simulink model "week3_inclass_ACC_v_1_1"  (R2020b)
settings: Solver=FixedStepAuto  StartTime=0.0  StopTime=500  RelTol=1e-3
undefined symbols (not defined in the file or in its folder): sigbuilder_block
libraries: simulink x3, pid_lib x2
settings Model: Creator=anime  LastModifiedBy=anime

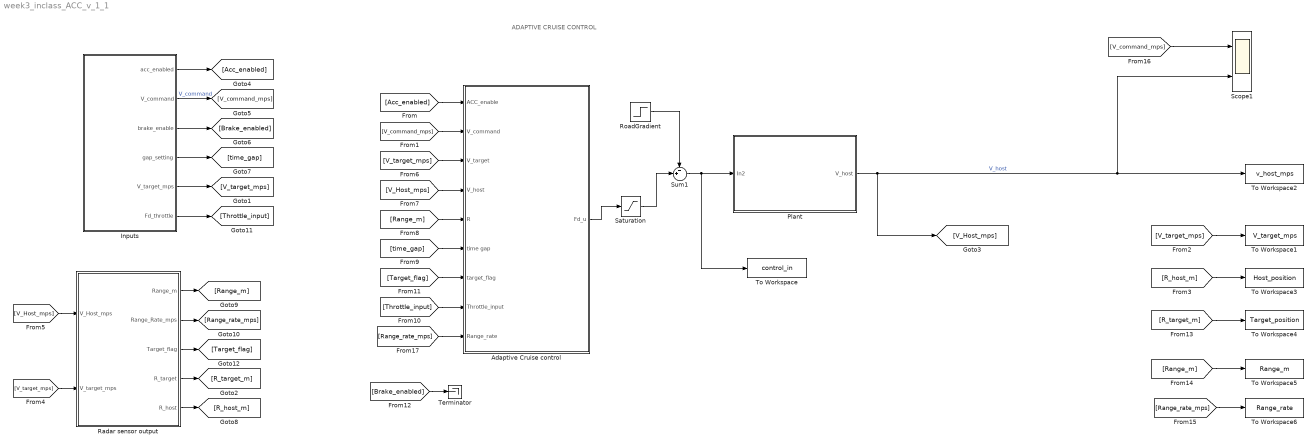
== system week3_inclass_ACC_v_1_1 ==
  note: ADAPTIVE CRUISE CONTROL
  Adaptive Cruise control : Subsystem
  Inputs : Subsystem
  Plant : Subsystem
  Radar sensor output : Subsystem
  RoadGradient : Step  Time=500  After=200  SampleTime=0
  Saturation : Saturate  UpperLimit=1000  LowerLimit=-1000
  Scope1 : Scope  NumInputPorts=2
  Sum1 : Sum  Inputs=-+|
  Terminator : Terminator
  To Workspace : ToWorkspace  VariableName=control_in  SampleTime=-1
  To Workspace1 : ToWorkspace  VariableName=V_target_mps  SampleTime=-1
  To Workspace2 : ToWorkspace  VariableName=v_host_mps  SampleTime=-1
  To Workspace3 : ToWorkspace  VariableName=Host_position  SampleTime=-1
  To Workspace4 : ToWorkspace  VariableName=Target_position  SampleTime=-1
  To Workspace5 : ToWorkspace  VariableName=Range_m  SampleTime=-1
  To Workspace6 : ToWorkspace  VariableName=Range_rate  SampleTime=-1
  wires:
  Adaptive Cruise control/1(Fd_u) -> Saturation/1
  Saturation/1 -> Sum1/2
  RoadGradient/1 -> Sum1/1
  Sum1/1 -> Plant/1(In2), To Workspace/1
  Plant/1(V_host) -> [V_Host_mps], Scope1/2, To Workspace2/1  "V_host"
  Inputs/1(acc_enabled) -> [Acc_enabled]
  Inputs/2(V_command) -> [V_command_mps]  "V_command"
  Inputs/6(Fd_throttle) -> [Throttle_input]
  Inputs/5(V_target_mps) -> [V_target_mps]
  Inputs/4(gap_setting) -> [time_gap]
  Inputs/3(brake_enable) -> [Brake_enabled]
  [V_command_mps] -> Adaptive Cruise control/2(V_command)
  [V_target_mps] -> Adaptive Cruise control/3(V_target)
  [V_Host_mps] -> Adaptive Cruise control/4(V_host)
  [time_gap] -> Adaptive Cruise control/6(time gap)
  [V_Host_mps] -> Radar sensor output/1(V_Host_mps)
  [V_target_mps] -> Radar sensor output/2(V_target_mps)
  Radar sensor output/1(Range_m) -> [Range_m]
  Radar sensor output/2(Range_Rate_mps) -> [Range_rate_mps]
  Radar sensor output/3(Target_flag) -> [Target_flag]
  [Range_m] -> Adaptive Cruise control/5(R)
  [Acc_enabled] -> Adaptive Cruise control/1(ACC_enable)
  [Target_flag] -> Adaptive Cruise control/7(target_flag)
  [Throttle_input] -> Adaptive Cruise control/8(Throttle_input)
  [Brake_enabled] -> Terminator/1
  Radar sensor output/4(R_target) -> [R_target_m]
  Radar sensor output/5(R_host) -> [R_host_m]
  [V_target_mps] -> To Workspace1/1
  [R_host_m] -> To Workspace3/1
  [R_target_m] -> To Workspace4/1
  [Range_m] -> To Workspace5/1
  [Range_rate_mps] -> To Workspace6/1
  [V_command_mps] -> Scope1/1
  [Range_rate_mps] -> Adaptive Cruise control/9(Range_rate)

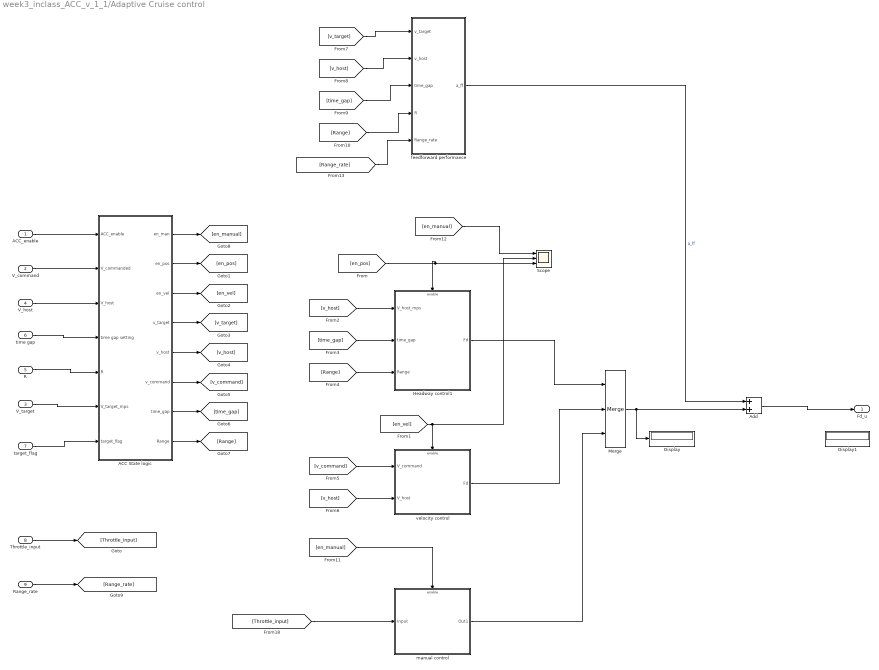
== system week3_inclass_ACC_v_1_1/Adaptive Cruise control ==
  ACC_enable : Inport
  V_command : Inport  Port=2
  V_target : Inport  Port=3
  V_host : Inport  Port=4
  R : Inport  Port=5
  time gap : Inport  Port=6
  target_flag : Inport  Port=7
  Throttle_input : Inport  Port=8
  Range_rate : Inport  Port=9
  ACC State logic : Subsystem
  Add : Sum
  Display : Display
  Display1 : Display
  Headway control1 : Subsystem
  Merge : Merge  Inputs=3
  Scope : Scope  NumInputPorts=3
  feedforward performance : Subsystem
  manual control : Subsystem
  velocity control : Subsystem
  Fd_u : Outport
  wires:
  [en_pos] -> Headway control1/Enable, Scope/3
  [en_vel] -> velocity control/Enable, Scope/2
  [time_gap] -> Headway control1/2(time_gap)
  [Range] -> Headway control1/3(Range)
  [v_command] -> velocity control/1(V_command)
  [v_host] -> velocity control/2(V_host)
  Headway control1/1(Fd) -> Merge/1
  velocity control/1(Fd) -> Merge/2
  [en_manual] -> manual control/Enable
  manual control/1(Out1) -> Merge/3
  [en_manual] -> Scope/1
  [Throttle_input] -> manual control/1(Input)
  ACC State logic/5(v_host) -> [v_host]
  ACC State logic/6(v_command) -> [v_command]
  ACC State logic/4(v_target) -> [v_target]
  ACC State logic/8(Range) -> [Range]
  V_host/1 -> ACC State logic/3(V_host)
  ACC State logic/7(time_gap) -> [time_gap]
  V_command/1 -> ACC State logic/2(V_commanded)
  R/1 -> ACC State logic/5(R)
  ACC_enable/1 -> ACC State logic/1(ACC_enable)
  ACC State logic/1(en_man) -> [en_manual]
  ACC State logic/2(en_pos) -> [en_pos]
  V_target/1 -> ACC State logic/6(V_target_mps)
  ACC State logic/3(en_vel) -> [en_vel]
  time gap/1 -> ACC State logic/4(time gap setting)
  target_flag/1 -> ACC State logic/7(target_flag)
  Throttle_input/1 -> [Throttle_input]
  [v_host] -> Headway control1/1(V_host_mps)
  Merge/1 -> Add/2, Display/1
  Range_rate/1 -> [Range_rate]
  Add/1 -> Fd_u/1
  [v_target] -> feedforward performance/1(v_target)
  [Range_rate] -> feedforward performance/5(Range_rate)
  [v_host] -> feedforward performance/2(v_host)
  [time_gap] -> feedforward performance/3(time_gap)
  [Range] -> feedforward performance/4(R)
  feedforward performance/1(a_ff) -> Add/1  "a_ff"

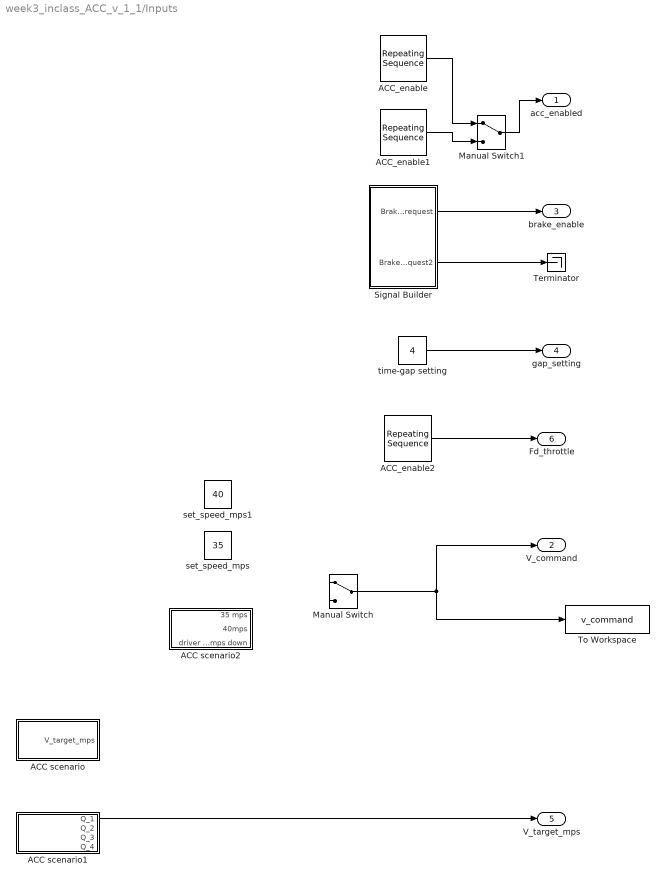
== system week3_inclass_ACC_v_1_1/Inputs ==
  ACC scenario : Subsystem  Tag=STV Subsys  LoadFcn=sigbuilder_block('load');  StartFcn=sigbuilder_block('start');  StopFcn=sigbuilder_block('stop');  ClipboardFcn=sigbuilder_block('clipboard');  mask(Sigbuilder block){tuvar=[0:10]}
      mask help: Simulink:masks:SigbuilderBlock_MD
      mask init:
      | if ~strcmp(get_param(bdroot(gcbh),'SimulationStatus'),'stopped') tuvar = sigbuilder_block('maskInit'); end
      settings: CopyFcn=sigbuilder_block('copy');  DeleteFcn=sigbuilder_block('delete');  ModelCloseFcn=sigbuilder_block('modelClose');  PreSaveFcn=sigbuilder_block('preSave');  PauseFcn=sigbuilder_block('pause');  ContinueFcn=sigbuilder_block('continue');  NameChangeFcn=sigbuilder_block('namechange');  OpenFcn=sigbuilder_block('open',[5.4 44.4 1141.2 541.8 ]);  CloseFcn=sigbuilder_block('close');
      mask Display: plot(0, 0, 100, 100,[2, 2, 32, 32, 2], [68, 8, 8, 68, 68],[32, 2], [38, 38], [32, 19, 2],[53, 60, 44], [32, 17, 17, 2],[16, 16, 31, 31]);txt = getActiveGroup(gcbh);text(2, 100, txt,'verticalAlignment', 'top');
  ACC scenario1 : Subsystem  Tag=STV Subsys  LoadFcn=sigbuilder_block('load');  StartFcn=sigbuilder_block('start');  StopFcn=sigbuilder_block('stop');  ClipboardFcn=sigbuilder_block('clipboard');  mask(Sigbuilder block){tuvar=[0:10]}
      mask help: Simulink:masks:SigbuilderBlock_MD
      mask init:
      | if ~strcmp(get_param(bdroot(gcbh),'SimulationStatus'),'stopped') tuvar = sigbuilder_block('maskInit'); end
      settings: CopyFcn=sigbuilder_block('copy');  DeleteFcn=sigbuilder_block('delete');  ModelCloseFcn=sigbuilder_block('modelClose');  PreSaveFcn=sigbuilder_block('preSave');  PauseFcn=sigbuilder_block('pause');  ContinueFcn=sigbuilder_block('continue');  NameChangeFcn=sigbuilder_block('namechange');  OpenFcn=sigbuilder_block('open',[12.75 109.5 1141.5 542.25 ]);  CloseFcn=sigbuilder_block('close');
      mask Display: plot(0, 0, 100, 100,[2, 2, 32, 32, 2], [68, 8, 8, 68, 68],[32, 2], [38, 38], [32, 19, 2],[53, 60, 44], [32, 17, 17, 2],[16, 16, 31, 31]);txt = getActiveGroup(gcbh);text(2, 100, txt,'verticalAlignment', 'top');
  ACC scenario2 : Subsystem  Tag=STV Subsys  LoadFcn=sigbuilder_block('load',[5.4 44.4 1141.2 541.8 ]);  StartFcn=sigbuilder_block('start');  StopFcn=sigbuilder_block('stop');  ClipboardFcn=sigbuilder_block('clipboard');  mask(Sigbuilder block){tuvar=[0:10]}
      mask help: Simulink:masks:SigbuilderBlock_MD
      mask init:
      | if ~strcmp(get_param(bdroot(gcbh),'SimulationStatus'),'stopped') tuvar = sigbuilder_block('maskInit'); end
      settings: CopyFcn=sigbuilder_block('copy');  DeleteFcn=sigbuilder_block('delete');  ModelCloseFcn=sigbuilder_block('modelClose');  PreSaveFcn=sigbuilder_block('preSave');  PauseFcn=sigbuilder_block('pause');  ContinueFcn=sigbuilder_block('continue');  NameChangeFcn=sigbuilder_block('namechange');  OpenFcn=sigbuilder_block('open',[5.4 44.4 1141.2 541.8 ]);  CloseFcn=sigbuilder_block('close');
      mask Display: plot(0, 0, 100, 100,[2, 2, 32, 32, 2], [68, 8, 8, 68, 68],[32, 2], [38, 38], [32, 19, 2],[53, 60, 44], [32, 17, 17, 2],[16, 16, 31, 31]);txt = getActiveGroup(gcbh);text(2, 100, txt,'verticalAlignment', 'top');
  ACC_enable : simulink/Sources/Repeating Sequence  rep_seq_t=[0 25 50 75 100 125 150 175 200 250 300 350 400 450 500 550 600 650 700]  rep_seq_y=[1 1 1 1 1 1 1 1 1 1 1 1 1 1 1 1 1 1 1]
  ACC_enable1 : simulink/Sources/Repeating Sequence  rep_seq_t=[0 25 50 75 100 125 150 175 200 250 300 350 400 450 500 550 600 650 700]  rep_seq_y=[1 1 1 1 1 1 1 1 1 0 0 0 0 0 0 1 1 1 1]
  ACC_enable2 : simulink/Sources/Repeating Sequence  rep_seq_t=[0 25 50 75 100 125 150 175 200 250 300 350 400 450 500 550 600 650 700]  rep_seq_y=[1 1 1 1 1 1 1 1 1 1 1 1 1 1 1 1 1 1 1]*0
  Manual Switch : ManualSwitch
  Manual Switch1 : ManualSwitch
  Signal Builder : Subsystem  Tag=STV Subsys  LoadFcn=sigbuilder_block('load');  StartFcn=sigbuilder_block('start');  StopFcn=sigbuilder_block('stop');  ClipboardFcn=sigbuilder_block('clipboard');  mask(Sigbuilder block){tuvar=[0:10]}
      mask help: Simulink:masks:SigbuilderBlock_MD
      mask init:
      | if ~strcmp(get_param(bdroot(gcbh),'SimulationStatus'),'stopped') tuvar = sigbuilder_block('maskInit'); end
      settings: CopyFcn=sigbuilder_block('copy');  DeleteFcn=sigbuilder_block('delete');  ModelCloseFcn=sigbuilder_block('modelClose');  PreSaveFcn=sigbuilder_block('preSave');  PauseFcn=sigbuilder_block('pause');  ContinueFcn=sigbuilder_block('continue');  NameChangeFcn=sigbuilder_block('namechange');  OpenFcn=sigbuilder_block('open',[305.4 42.6 814.8 400.2 ]);  CloseFcn=sigbuilder_block('close');
      mask Display: plot(0, 0, 100, 100,[2, 2, 32, 32, 2], [68, 8, 8, 68, 68],[32, 2], [38, 38], [32, 19, 2],[53, 60, 44], [32, 17, 17, 2],[16, 16, 31, 31]);txt = getActiveGroup(gcbh);text(2, 100, txt,'verticalAlignment', 'top');
  Terminator : Terminator
  To Workspace : ToWorkspace  VariableName=v_command  SampleTime=-1
  set_speed_mps : Constant  Value=35
  set_speed_mps1 : Constant  Value=40
  time-gap setting : Constant  Value=4
  acc_enabled : Outport
  V_command : Outport  Port=2
  brake_enable : Outport  Port=3
  gap_setting : Outport  Port=4
  V_target_mps : Outport  Port=5
  Fd_throttle : Outport  Port=6
  wires:
  Signal Builder/1(Brake_request) -> brake_enable/1
  time-gap setting/1 -> gap_setting/1
  Signal Builder/2(Brake_request2) -> Terminator/1
  ACC_enable2/1 -> Fd_throttle/1
  Manual Switch/1 -> V_command/1, To Workspace/1
  ACC_enable/1 -> Manual Switch1/1
  Manual Switch1/1 -> acc_enabled/1
  ACC_enable1/1 -> Manual Switch1/2
  ACC scenario1/1(Q_1) -> V_target_mps/1

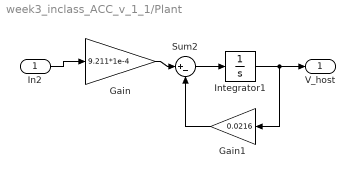
== system week3_inclass_ACC_v_1_1/Plant ==
  In2 : Inport
  Gain : Gain  Gain=9.211*1e-4
  Gain1 : Gain  Gain=0.0216
  Integrator1 : Integrator  InitialCondition=25
  Sum2 : Sum  Inputs=|+-
  V_host : Outport  VectorParamsAs1DForOutWhenUnconnected=off
  wires:
  Gain1/1 -> Sum2/2
  Integrator1/1 -> Gain1/1, V_host/1
  Gain/1 -> Sum2/1
  Sum2/1 -> Integrator1/1
  In2/1 -> Gain/1

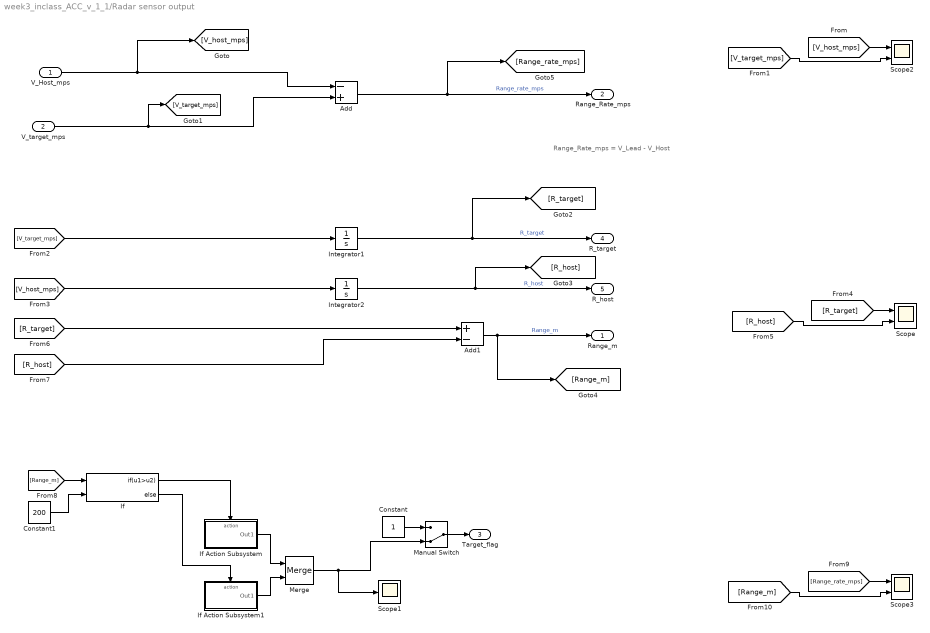
== system week3_inclass_ACC_v_1_1/Radar sensor output ==
  note: Range_Rate_mps = V_Lead - V_Host
  V_Host_mps : Inport
  V_target_mps : Inport  Port=2
  Add : Sum  Inputs=-+
  Add1 : Sum  Inputs=+-
  Constant : Constant
  Constant1 : Constant  Value=200
  If : If  NumInputs=2  IfExpression=u1>u2
  If Action Subsystem : Subsystem  TreatAsAtomicUnit=on
  If Action Subsystem1 : Subsystem  TreatAsAtomicUnit=on
  Integrator1 : Integrator  InitialCondition=500
  Integrator2 : Integrator
  Manual Switch : ManualSwitch  CurrentSetting=0
  Merge : Merge
  Scope : Scope  NumInputPorts=2
  Scope1 : Scope
  Scope2 : Scope  NumInputPorts=2
  Scope3 : Scope  NumInputPorts=2
  Range_m : Outport
  Range_Rate_mps : Outport  Port=2
  Target_flag : Outport  Port=3
  R_target : Outport  Port=4
  R_host : Outport  Port=5
  wires:
  V_target_mps/1 -> Add/2, [V_target_mps]
  V_Host_mps/1 -> Add/1, [V_host_mps]
  Add/1 -> [Range_rate_mps], Range_Rate_mps/1  "Range_rate_mps"
  Integrator1/1 -> [R_target], R_target/1  "R_target"
  Integrator2/1 -> [R_host], R_host/1  "R_host"
  Add1/1 -> [Range_m], Range_m/1  "Range_m"
  Constant/1 -> Manual Switch/1
  Manual Switch/1 -> Target_flag/1
  If/1 -> If Action Subsystem/Action
  If/2 -> If Action Subsystem1/Action
  If Action Subsystem/1(Out1) -> Merge/1
  If Action Subsystem1/1(Out1) -> Merge/2
  Merge/1 -> Scope1/1, Manual Switch/2
  Constant1/1 -> If/2
  [V_host_mps] -> Scope2/1
  [V_target_mps] -> Scope2/2
  [V_target_mps] -> Integrator1/1
  [V_host_mps] -> Integrator2/1
  [R_target] -> Scope/1
  [R_host] -> Scope/2
  [R_target] -> Add1/1
  [R_host] -> Add1/2
  [Range_m] -> If/1
  [Range_rate_mps] -> Scope3/1
  [Range_m] -> Scope3/2

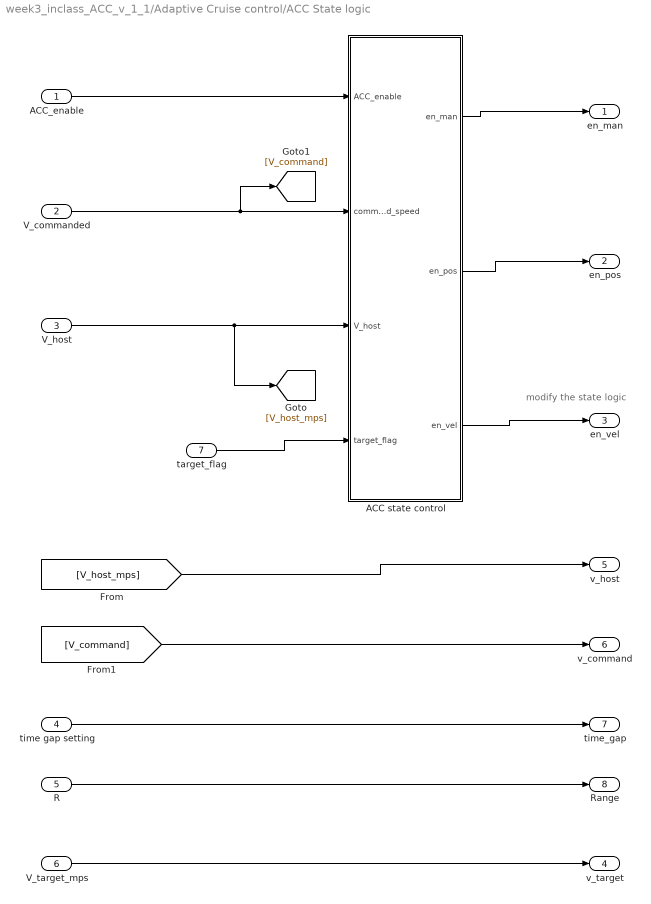
== system week3_inclass_ACC_v_1_1/Adaptive Cruise control/ACC State logic ==
  note: modify the state logic
  ACC_enable : Inport
  V_commanded : Inport  Port=2
  V_host : Inport  Port=3
  time gap setting : Inport  Port=4
  R : Inport  Port=5
  V_target_mps : Inport  Port=6
  target_flag : Inport  Port=7
  ACC state control : Stateflow chart  TreatAsAtomicUnit=on
  en_man : Outport
  en_pos : Outport  Port=2
  en_vel : Outport  Port=3
  v_target : Outport  Port=4
  v_host : Outport  Port=5
  v_command : Outport  Port=6
  time_gap : Outport  Port=7
  Range : Outport  Port=8
  wires:
  ACC state control/1(en_man) -> en_man/1
  ACC state control/2(en_pos) -> en_pos/1
  ACC state control/3(en_vel) -> en_vel/1
  ACC_enable/1 -> ACC state control/1(ACC_enable)
  V_commanded/1 -> [V_command], ACC state control/2(commanded_speed)
  V_target_mps/1 -> v_target/1
  V_host/1 -> [V_host_mps], ACC state control/3(V_host)
  target_flag/1 -> ACC state control/4(target_flag)
  [V_host_mps] -> v_host/1
  [V_command] -> v_command/1
  time gap setting/1 -> time_gap/1
  R/1 -> Range/1

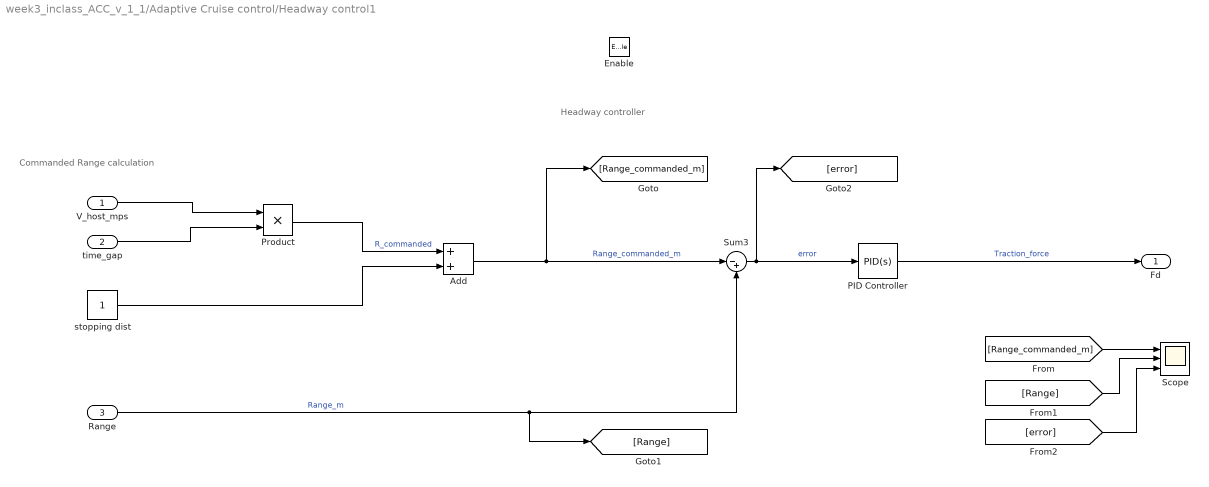
== system week3_inclass_ACC_v_1_1/Adaptive Cruise control/Headway control1 ==
  note: Commanded Range calculation
  note: Headway controller
  V_host_mps : Inport
  time_gap : Inport  Port=2
  Range : Inport  Port=3
  Enable : EnablePort
  Add : Sum
  PID Controller : pid_lib/PID Controller  Controller=PID  Form=Parallel  TimeDomain=Continuous-time  UseExternalTs=off  SampleTime=-1  IntegratorMethod=Forward Euler  FilterMethod=Forward Euler  ControllerParametersSource=internal  P=100  I=3  D=950  UseFilter=on  N=75  TunerSelectOption=Transfer Function Based (PID Tuner App)  InitialConditionSource=internal  InitialConditionForIntegrator=0  InitialConditionForFilter=0  DifferentiatorICPrevScaledInput=0  ExternalReset=none  TrackingMode=off  Kt=1  LimitOutput=off  SatLimitsSource=internal  UpperSaturationLimit=inf  LowerSaturationLimit=-inf  LinearizeAsGain=on  AntiWindupMode=none  Kb=1  POutMin=[]  POutMax=[]  IOutMin=[]  IOutMax=[]  DOutMin=[]  DOutMax=[]  NOutMin=[]  NOutMax=[]  SumOutMin=[]  SumOutMax=[]  SaturationOutMin=[]  SaturationOutMax=[]  PParamMin=[]  PParamMax=[]  IParamMin=[]  IParamMax=[]  DParamMin=[]  DParamMax=[]  NParamMin=[]  NParamMax=[]  KbParamMin=[]  KbParamMax=[]  KtParamMin=[]  KtParamMax=[]  KbOutMin=[]  KbOutMax=[]  KtOutMin=[]  KtOutMax=[]  IntegratorOutMin=[]  IntegratorOutMax=[]  FilterOutMin=[]  FilterOutMax=[]  SumI1OutMin=[]  SumI1OutMax=[]  SumI2OutMin=[]  SumI2OutMax=[]  SumI3OutMin=[]  SumI3OutMax=[]  SumI4OutMin=[]  SumI4OutMax=[]  SumDOutMin=[]  SumDOutMax=[]  DifferentiatorOutMin=[]  DifferentiatorOutMax=[]  FilterDiffOutCoefMin=[]  FilterDiffOutCoefMax=[]  ReciprocalOutMin=[]  ReciprocalOutMax=[]  SumDenOutMin=[]  SumDenOutMax=[]  SumNumOutMin=[]  SumNumOutMax=[]  DivideOutMin=[]  DivideOutMax=[]  UdiffTsProdOutMin=[]  UdiffTsProdOutMax=[]  NTsProdOutMin=[]  NTsProdOutMax=[]  UintegralTsProdOutMin=[]  UintegralTsProdOutMax=[]  UngainTsProdOutMin=[]  UngainTsProdOutMax=[]  IntegratorContinuousStateAttributes=''  IntegratorStateMustResolveToSignalObject=off  IntegratorRTWStateStorageClass=Auto  FilterContinuousStateAttributes=''  FilterStateMustResolveToSignalObject=off  FilterRTWStateStorageClass=Auto  ParallelPVariant=InternalParameters  IdealPVariant=Disabled  IVariant=InternalParameters  DVariant=InternalParameters  IntegratorVariant=Continuous  SatVariant=Disabled  AWVariant=Passthrough  PCopyVariant=Disabled  TRVariant=Disabled  FdbkBlocksVariant=Forward  IdealPFdbkVariant=Disabled  SatFdbkVariant=Disabled  DerivativeFilterVariant=ContFilter  NVariant=InternalParameters  NCopyVariant=Disabled  FilterICVariant=InternalICsFilter  IntegratorICVariant=InternalICs  ExternalResetVariant=Disabled  TRSumVariant=Passthrough  SumFdbkVariant=Disabled  SumVariant=Sum_PID  TsampFilterVariant=InternalTs  TsampNgainVariant=Passthrough  TsampIntegralVariant=Passthrough  ExternalSaturationOutDataTypeStr=Inherit: Same as second input
  Product : Product
  Scope : Scope  NumInputPorts=3
  Sum3 : Sum  Inputs=|-+
  stopping dist : Constant
  Fd : Outport
  wires:
  stopping dist/1 -> Add/2
  PID Controller/1 -> Fd/1  "Traction_force"
  Product/1 -> Add/1  "R_commanded"
  time_gap/1 -> Product/2
  Add/1 -> [Range_commanded_m], Sum3/1  "Range_commanded_m"
  Range/1 -> [Range], Sum3/2  "Range_m"
  [Range] -> Scope/2
  [Range_commanded_m] -> Scope/1
  Sum3/1 -> [error], PID Controller/1  "error"
  [error] -> Scope/3
  V_host_mps/1 -> Product/1

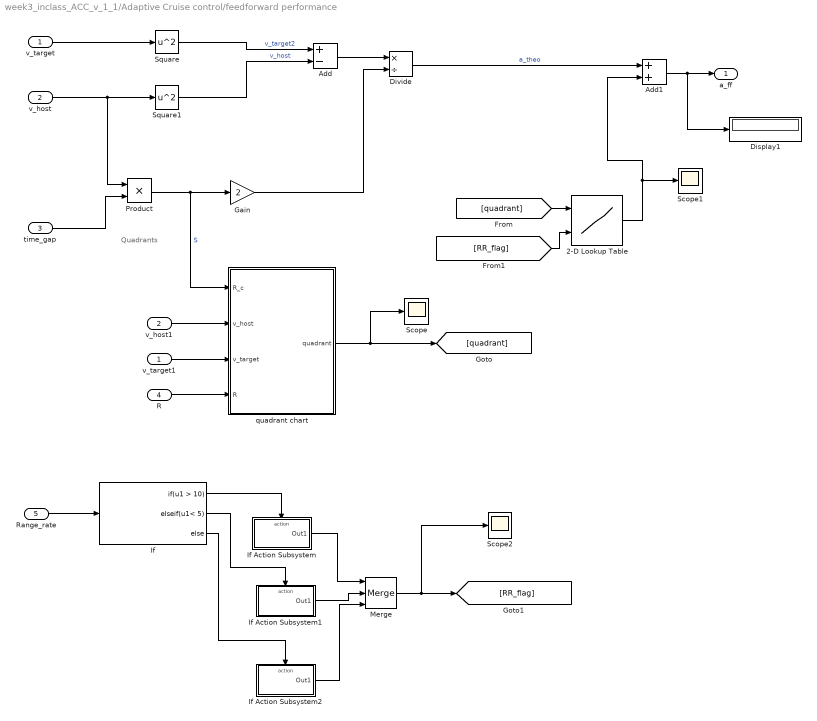
== system week3_inclass_ACC_v_1_1/Adaptive Cruise control/feedforward performance ==
  note: Quadrants
  v_target : Inport
  v_host : Inport  Port=2
  time_gap : Inport  Port=3
  R : Inport  Port=4
  Range_rate : Inport  Port=5
  2-D Lookup Table : Lookup_n-D  BreakpointsForDimension1=[1,2,3,4]  BreakpointsForDimension2=[1,2,3]  Table=reshape([10,15,10,20,30,19,18,38,50,20,23,43],4,3)  InternalRulePriority=Speed  RndMeth=Simplest  InputSameDT=on
      settings: InputPortMap=u0,u1
  Add : Sum  Inputs=+-
  Add1 : Sum
  Display1 : Display
  Divide : Product  Inputs=*/
  Gain : Gain  Gain=2
  If : If  IfExpression=u1 > 10  ElseIfExpressions=u1< 5
  If Action Subsystem : Subsystem  TreatAsAtomicUnit=on
  If Action Subsystem1 : Subsystem  TreatAsAtomicUnit=on
  If Action Subsystem2 : Subsystem  TreatAsAtomicUnit=on
  Merge : Merge  Inputs=3
  Product : Product
  Scope : Scope
  Scope1 : Scope
  Scope2 : Scope
  Square : Math  Operator=square  SaturateOnIntegerOverflow=on
  Square1 : Math  Operator=square  SaturateOnIntegerOverflow=on
  quadrant chart : Stateflow chart  TreatAsAtomicUnit=on
  v_host1 : InportShadow  Port=2
  v_target1 : InportShadow
  a_ff : Outport
  wires:
  v_target/1 -> Square/1
  Square/1 -> Add/1  "v_target2"
  Square1/1 -> Add/2  "v_host"
  Add/1 -> Divide/1
  time_gap/1 -> Product/2
  Product/1 -> quadrant chart/1(R_c), Gain/1  "S"
  Gain/1 -> Divide/2
  v_host1/1 -> quadrant chart/2(v_host)
  v_target1/1 -> quadrant chart/3(v_target)
  R/1 -> quadrant chart/4(R)
  quadrant chart/1(quadrant) -> Scope/1, [quadrant]
  [quadrant] -> 2-D Lookup Table/1
  Add1/1 -> Display1/1, a_ff/1
  2-D Lookup Table/1 -> Scope1/1, Add1/2
  Divide/1 -> Add1/1  "a_theo"
  v_host/1 -> Product/1, Square1/1
  Range_rate/1 -> If/1
  [RR_flag] -> 2-D Lookup Table/2
  Merge/1 -> Scope2/1, [RR_flag]
  If/1 -> If Action Subsystem/Action
  If/2 -> If Action Subsystem1/Action
  If/3 -> If Action Subsystem2/Action
  If Action Subsystem/1(Out1) -> Merge/1
  If Action Subsystem1/1(Out1) -> Merge/2
  If Action Subsystem2/1(Out1) -> Merge/3

== system week3_inclass_ACC_v_1_1/Adaptive Cruise control/manual control ==
  Input : Inport
  Enable : EnablePort
  Out1 : Outport
  wires:
  Input/1 -> Out1/1

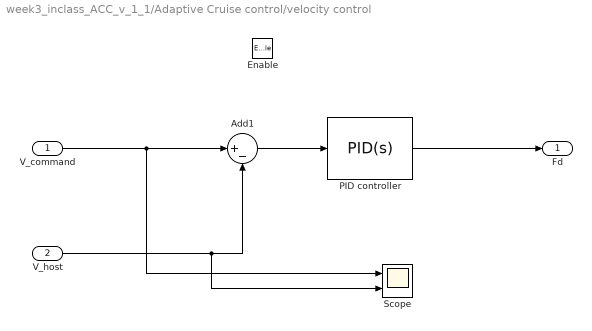
== system week3_inclass_ACC_v_1_1/Adaptive Cruise control/velocity control ==
  V_command : Inport
  V_host : Inport  Port=2
  Enable : EnablePort
  Add1 : Sum  Inputs=|+-
  PID controller : pid_lib/PID Controller  Controller=PID  Form=Parallel  TimeDomain=Continuous-time  UseExternalTs=off  SampleTime=-1  IntegratorMethod=Forward Euler  FilterMethod=Forward Euler  ControllerParametersSource=internal  P=350  I=8.132  D=0  UseFilter=on  N=75  TunerSelectOption=Transfer Function Based (PID Tuner App)  InitialConditionSource=internal  InitialConditionForIntegrator=0  InitialConditionForFilter=0  DifferentiatorICPrevScaledInput=0  ExternalReset=none  TrackingMode=off  Kt=1  LimitOutput=off  SatLimitsSource=internal  UpperSaturationLimit=inf  LowerSaturationLimit=-inf  LinearizeAsGain=on  AntiWindupMode=none  Kb=1  POutMin=[]  POutMax=[]  IOutMin=[]  IOutMax=[]  DOutMin=[]  DOutMax=[]  NOutMin=[]  NOutMax=[]  SumOutMin=[]  SumOutMax=[]  SaturationOutMin=[]  SaturationOutMax=[]  PParamMin=[]  PParamMax=[]  IParamMin=[]  IParamMax=[]  DParamMin=[]  DParamMax=[]  NParamMin=[]  NParamMax=[]  KbParamMin=[]  KbParamMax=[]  KtParamMin=[]  KtParamMax=[]  KbOutMin=[]  KbOutMax=[]  KtOutMin=[]  KtOutMax=[]  IntegratorOutMin=[]  IntegratorOutMax=[]  FilterOutMin=[]  FilterOutMax=[]  SumI1OutMin=[]  SumI1OutMax=[]  SumI2OutMin=[]  SumI2OutMax=[]  SumI3OutMin=[]  SumI3OutMax=[]  SumI4OutMin=[]  SumI4OutMax=[]  SumDOutMin=[]  SumDOutMax=[]  DifferentiatorOutMin=[]  DifferentiatorOutMax=[]  FilterDiffOutCoefMin=[]  FilterDiffOutCoefMax=[]  ReciprocalOutMin=[]  ReciprocalOutMax=[]  SumDenOutMin=[]  SumDenOutMax=[]  SumNumOutMin=[]  SumNumOutMax=[]  DivideOutMin=[]  DivideOutMax=[]  UdiffTsProdOutMin=[]  UdiffTsProdOutMax=[]  NTsProdOutMin=[]  NTsProdOutMax=[]  UintegralTsProdOutMin=[]  UintegralTsProdOutMax=[]  UngainTsProdOutMin=[]  UngainTsProdOutMax=[]  IntegratorContinuousStateAttributes=''  IntegratorStateMustResolveToSignalObject=off  IntegratorRTWStateStorageClass=Auto  FilterContinuousStateAttributes=''  FilterStateMustResolveToSignalObject=off  FilterRTWStateStorageClass=Auto  ParallelPVariant=InternalParameters  IdealPVariant=Disabled  IVariant=InternalParameters  DVariant=InternalParameters  IntegratorVariant=Continuous  SatVariant=Disabled  AWVariant=Passthrough  PCopyVariant=Disabled  TRVariant=Disabled  FdbkBlocksVariant=Forward  IdealPFdbkVariant=Disabled  SatFdbkVariant=Disabled  DerivativeFilterVariant=ContFilter  NVariant=InternalParameters  NCopyVariant=Disabled  FilterICVariant=InternalICsFilter  IntegratorICVariant=InternalICs  ExternalResetVariant=Disabled  TRSumVariant=Passthrough  SumFdbkVariant=Disabled  SumVariant=Sum_PID  TsampFilterVariant=InternalTs  TsampNgainVariant=Passthrough  TsampIntegralVariant=Passthrough  ExternalSaturationOutDataTypeStr=Inherit: Same as second input
  Scope : Scope  NumInputPorts=2
  Fd : Outport
  wires:
  Add1/1 -> PID controller/1
  V_command/1 -> Scope/1, Add1/1
  PID controller/1 -> Fd/1
  V_host/1 -> Scope/2, Add1/2

== system week3_inclass_ACC_v_1_1/Inputs/ACC scenario ==
  Demux : Demux  Tag=STV Demux  Outputs=1
      settings: DisplayOption=none
  FromWs : FromWorkspace  Tag=STV FromWs  VariableName=tuvar
      SigBuilderData=|
      | common.afterFinalStr = 'Extrapolate'
      | common.sampleTime = 0
      | dataSet.timeRange = [0 500]
      | dataSet.name = 'Group 1'
      | sbobj.Groups.Name = 'Group 1'
      | sbobj.Groups.Signals.Name = 'V_target_mps'
      | sbobj.Groups.Signals.XData = [0 4 212.5 212.5 339.5 399.5 399.5 500]
      | sbobj.Groups.Signals.YData = [34.8 35 35 28.65 28.65 28.65 37.7 37.7]
      | sbobj.Groups.TimeRange = [0 500]
  V_target_mps : Outport  Tag=STV Outport
  wires:
  Demux/1 -> V_target_mps/1
  FromWs/1 -> Demux/1

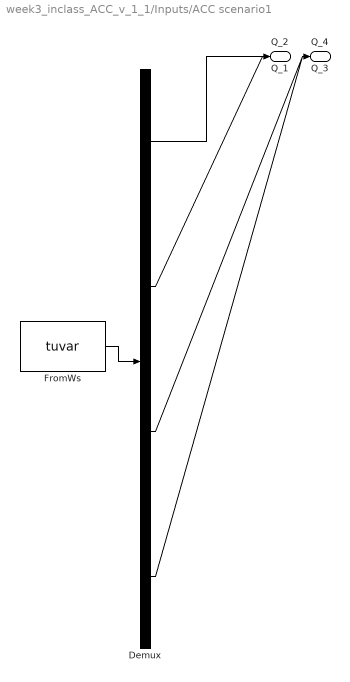
== system week3_inclass_ACC_v_1_1/Inputs/ACC scenario1 ==
  Demux : Demux  Tag=STV Demux
      settings: DisplayOption=none
  FromWs : FromWorkspace  Tag=STV FromWs  VariableName=tuvar
      SigBuilderData=|
      | common.afterFinalStr = 'Extrapolate'
      | common.sampleTime = 0
      | dataSet.timeRange = [0 500]
      | dataSet.name = 'Group 1'
      | sbobj.Groups.Name = 'Group 1'
      | sbobj.Groups.Signals(1).Name = 'Q_1'
      | sbobj.Groups.Signals(1).XData = [0 500]
      | sbobj.Groups.Signals(1).YData = [45 45]
      | sbobj.Groups.Signals(2).Name = 'Q_2'
      | sbobj.Groups.Signals(2).XData = [0 300.5 300.5 500]
      | sbobj.Groups.Signals(2).YData = [0 0 28 28]
      | sbobj.Groups.Signals(3).Name = 'Q_3'
      | sbobj.Groups.Signals(3).XData = [0 250 250 500]
      | sbobj.Groups.Signals(3).YData = [25 25 9.8 9.8]
      | sbobj.Groups.Signals(4).Name = 'Q_4'
      | sbobj.Groups.Signals(4).XData = [0 250 250 500]
      | sbobj.Groups.Signals(4).YData = [25 25 40 40]
      | sbobj.Groups.TimeRange = [0 500]
  Q_1 : Outport  Tag=STV Outport
  Q_2 : Outport  Tag=STV Outport  Port=2
  Q_3 : Outport  Tag=STV Outport  Port=3
  Q_4 : Outport  Tag=STV Outport  Port=4
  wires:
  FromWs/1 -> Demux/1
  Demux/1 -> Q_1/1
  Demux/2 -> Q_2/1
  Demux/3 -> Q_3/1
  Demux/4 -> Q_4/1

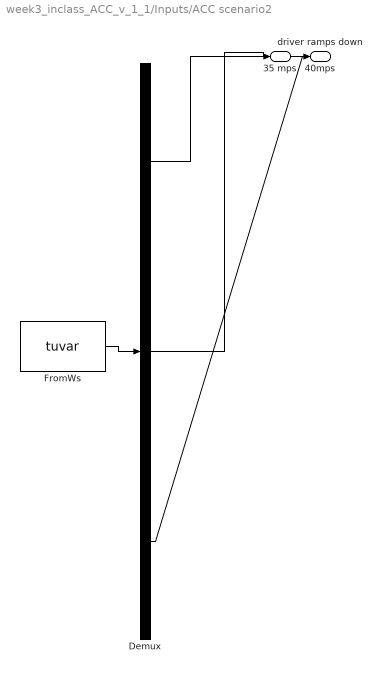
== system week3_inclass_ACC_v_1_1/Inputs/ACC scenario2 ==
  Demux : Demux  Tag=STV Demux  Outputs=3
      settings: DisplayOption=none
  FromWs : FromWorkspace  Tag=STV FromWs  VariableName=tuvar
      SigBuilderData=|
      | common.afterFinalStr = 'Extrapolate'
      | common.sampleTime = 0
      | dataSet.timeRange = [0 500]
      | dataSet.name = 'Group 1'
      | sbobj.Groups.Name = 'Group 1'
      | sbobj.Groups.Signals(1).Name = '35 mps'
      | sbobj.Groups.Signals(1).XData = [0 500]
      | sbobj.Groups.Signals(1).YData = [35 35]
      | sbobj.Groups.Signals(2).Name = '40mps'
      | sbobj.Groups.Signals(2).XData = [0 500]
      | sbobj.Groups.Signals(2).YData = [40 40]
      | sbobj.Groups.Signals(3).Name = 'driver ramps down '
      | sbobj.Groups.Signals(3).XData = [0 99.5 99.5 106 106 112.5 112.5 119 119 125.5 125.5 133 133 500]
      | sbobj.Groups.Signals(3).YData = [35 35 34 34 32 32 30 30 28 28 26 26 25 25]
      | sbobj.Groups.TimeRange = [0 500]
  35 mps : Outport  Tag=STV Outport
  40mps : Outport  Tag=STV Outport  Port=2
  "driver ramps down " : Outport  Tag=STV Outport  Port=3
  wires:
  FromWs/1 -> Demux/1
  Demux/1 -> 35 mps/1
  Demux/2 -> 40mps/1
  Demux/3 -> "driver ramps down "/1

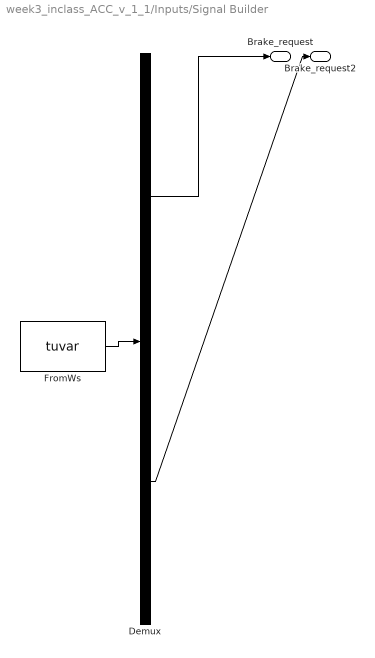
== system week3_inclass_ACC_v_1_1/Inputs/Signal Builder ==
  Demux : Demux  Tag=STV Demux  Outputs=2
      settings: DisplayOption=none
  FromWs : FromWorkspace  Tag=STV FromWs  VariableName=tuvar
      SigBuilderData=|
      | common.afterFinalStr = 'Extrapolate'
      | common.sampleTime = 0
      | dataSet.timeRange = [0 700]
      | dataSet.name = 'Group 1'
      | sbobj.Groups.Name = 'Group 1'
      | sbobj.Groups.Signals(1).Name = 'Brake_request'
      | sbobj.Groups.Signals(1).XData = [0 4 6 700]
      | sbobj.Groups.Signals(1).YData = [0 0 0 0]
      | sbobj.Groups.Signals(2).Name = 'Brake_request2'
      | sbobj.Groups.Signals(2).XData = [0 340 340 700]
      | sbobj.Groups.Signals(2).YData = [0 0 1 1]
      | sbobj.Groups.TimeRange = [0 700]
  Brake_request : Outport  Tag=STV Outport
  Brake_request2 : Outport  Tag=STV Outport  Port=2
  wires:
  Demux/1 -> Brake_request/1
  FromWs/1 -> Demux/1
  Demux/2 -> Brake_request2/1

== system week3_inclass_ACC_v_1_1/Radar sensor output/If Action Subsystem ==
  Action Port : ActionPort  ActionPortLabel=if(u1>u2)
  Constant : Constant  Value=0
  Out1 : Outport
  wires:
  Constant/1 -> Out1/1

== system week3_inclass_ACC_v_1_1/Radar sensor output/If Action Subsystem1 ==
  Action Port : ActionPort  ActionPortLabel=else
  Constant : Constant
  Out1 : Outport
  wires:
  Constant/1 -> Out1/1

== system week3_inclass_ACC_v_1_1/Adaptive Cruise control/feedforward performance/If Action Subsystem ==
  Action Port : ActionPort  ActionPortLabel=if(u1 > 10)
  Constant : Constant
  Out1 : Outport
  wires:
  Constant/1 -> Out1/1

== system week3_inclass_ACC_v_1_1/Adaptive Cruise control/feedforward performance/If Action Subsystem1 ==
  Action Port : ActionPort  ActionPortLabel=elseif(u1< 5)
  Constant : Constant  Value=3
  Out1 : Outport
  wires:
  Constant/1 -> Out1/1

== system week3_inclass_ACC_v_1_1/Adaptive Cruise control/feedforward performance/If Action Subsystem2 ==
  Action Port : ActionPort  ActionPortLabel=else
  Constant : Constant  Value=2
  Out1 : Outport
  wires:
  Constant/1 -> Out1/1

== stateflow chart week3_inclass_ACC_v_1_1/Adaptive Cruise control/feedforward performance/quadrant chart ==
  state quadrant2
    entry:
    quadrant  = 2;
  state quadrant1
    entry:
    quadrant  = 1;
  state quadrant4
    entry:
    quadrant  = 4;
  state quadrant3
    entry:
    quadrant  = 3;
  (default) -> quadrant1
  quadrant1 -> (junction 7) : [((R<R_c) || (v_target< v_host))&& after(10,sec)]
  (junction 7) -> quadrant2 [order 4] : [(R>R_c)&&(v_target < v_host)]
  quadrant2 -> (junction 7) : [((R>R_c) || (v_target> v_host))&& after(10,sec)]
  (junction 7) -> quadrant1 [order 1] : [(R>R_c)&&(v_target > v_host) ]
  quadrant3 -> (junction 7) : [((R>R_c) || (v_target> v_host)&& after(10,sec))]
  (junction 7) -> quadrant3 [order 3] : [(R<R_c)&&(v_target < v_host)]
  quadrant4 -> (junction 7) : [((R>R_c) || (v_target< v_host))&& after(10,sec)]
  (junction 7) -> quadrant4 [order 2] : [(R<R_c)&&(v_target > v_host) ]
  data: R_c input; v_host input; v_target input; quadrant output; R input

== stateflow chart week3_inclass_ACC_v_1_1/Adaptive Cruise control/ACC State logic/ACC state control ==
  state HeadwayControl
    entry: en_man=false;
    en_vel = false;
    en_pos = true;
  state Manual__
    entry: en_man=true;
    en_vel = false;
    en_pos = false;
  state VelocityControl_
    entry: en_man=false ;
    en_vel = true;
    en_pos = false;
  Manual__ -> VelocityControl_ [order 1] : [(ACC_enable==1) &(target_flag==0)]
  Manual__ -> HeadwayControl [order 2] : [(ACC_enable==1) &(target_flag==1)]
  VelocityControl_ -> HeadwayControl [order 2] : [(ACC_enable==1) &(target_flag==1)&& after(30,sec) ]
  (default) -> Manual__
  VelocityControl_ -> Manual__ [order 1] : [(ACC_enable==0) ]
  HeadwayControl -> VelocityControl_ [order 2] : [((ACC_enable==1) &(target_flag==0) || V_host >commanded_speed+0.5) &&  after(20,sec) ]
  HeadwayControl -> Manual__ [order 1] : [(ACC_enable==0) ]
  data: en_man output; en_pos output; en_vel output; ACC_enable input; commanded_speed input; V_host input; target_flag input
